simulink model "pendel_kartesisch"  (Simulink 7.0)
settings: Solver=ode45  StartTime=0.0  StopTime=tstop  FixedStep=0.3  MaxStep=0.25  RelTol=1e-6
values from neighbouring files (symbols this model uses):
  g = 9.81    [main_pendel_kartesisch.m]    (also in main_pendel_polar.m)
  l = 1    [main_pendel_kartesisch.m]    (also in main_pendel_polar.m)
  lamda_t0 = (vx0^2 + vy0^2 -g*y0)/(l^2)    [main_pendel_kartesisch.m]
  x0 = 1    [main_pendel_kartesisch.m]
  y0 = -sqrt(l^2-x0^2)    [main_pendel_kartesisch.m]
libraries: simulink x5
settings Model: Creator=adminus  LastModifiedBy=adminus
settings DataIOCC: OutputOption=SpecifiedOutputTimes  OutputTimes=[0:0.01:5]
settings OptimizationCC: BlockReduction=off
settings DebuggingCC: SaveWithParameterizedLinksMsg=none  SignalResolutionControl=TryResolveAllWithWarning  SolverPrmCheckMsg=none  MultiTaskDSMMsg=warning  MultiTaskCondExecSysMsg=none  StrictBusMsg=None
settings HardwareCC: TargetUnknown=on
settings RTWCC: IncludeERTFirstTime=on

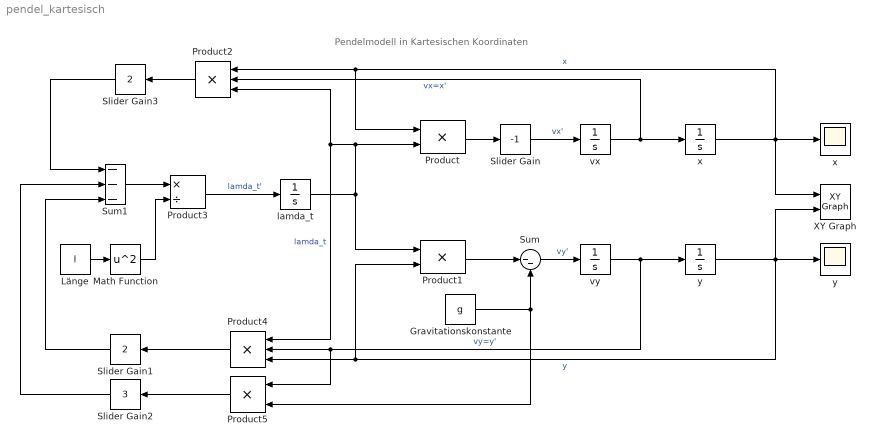
== system pendel_kartesisch ==
  note: Pendelmodell in Kartesischen Koordinaten
  Gravitationskonstante : Constant  Value=g
  Länge : Constant  Value=l
  Math Function : Math  Operator=square  SaturateOnIntegerOverflow=on
  Product : Product  SaturateOnIntegerOverflow=on  RndMeth=Zero  InputSameDT=on
  Product1 : Product  SaturateOnIntegerOverflow=on  RndMeth=Zero  InputSameDT=on
  Product2 : Product  Orientation=left  Inputs=3  SaturateOnIntegerOverflow=on  RndMeth=Zero  InputSameDT=on
  Product3 : Product  Inputs=*/  SaturateOnIntegerOverflow=on  RndMeth=Zero  InputSameDT=on
  Product4 : Product  Orientation=left  Inputs=3  SaturateOnIntegerOverflow=on  RndMeth=Zero  InputSameDT=on
  Product5 : Product  Orientation=left  SaturateOnIntegerOverflow=on  RndMeth=Zero  InputSameDT=on
  Slider Gain : simulink/Math Operations/Slider Gain  SystemSampleTime=-1  low=-1  gain=-1  high=2
  Slider Gain1 : simulink/Math Operations/Slider Gain  Orientation=left  SystemSampleTime=-1  low=-1  gain=2  high=2
  Slider Gain2 : simulink/Math Operations/Slider Gain  Orientation=left  SystemSampleTime=-1  low=-1  gain=3  high=3
  Slider Gain3 : simulink/Math Operations/Slider Gain  Orientation=left  SystemSampleTime=-1  low=-1  gain=2  high=2
  Sum : Sum  Inputs=|--  SaturateOnIntegerOverflow=on  InputSameDT=on
  Sum1 : Sum  Inputs=---  SaturateOnIntegerOverflow=on  InputSameDT=on
  XY Graph : simulink/Sinks/XY Graph  SystemSampleTime=-1  xmin=-1.1*l  xmax=1.1*l  ymin=-1.1*l  ymax=1.1*l  st=-1
  lamda_t : Integrator  InitialCondition=lamda_t0
  vx : Integrator
  vy : Integrator
  x : Scope
      settings: SaveName=ScopeData_v1_x
  "x " : Integrator  InitialCondition=x0
  y : Scope
      settings: SaveName=ScopeData_v1_y
  "y " : Integrator  InitialCondition=y0
  wires:
  lamda_t/1 -> Product/2, Product2/3, Product4/1, Product1/1  "lamda_t"
  Product1/1 -> Sum/1
  Slider Gain/1 -> vx/1  "vx'"
  Sum/1 -> vy/1  "vy'"
  Gravitationskonstante/1 -> Sum/2, Product5/2
  Sum1/1 -> Product3/1
  Länge/1 -> Math Function/1
  Product4/1 -> Slider Gain1/1
  Product2/1 -> Slider Gain3/1
  Product5/1 -> Slider Gain2/1
  Slider Gain1/1 -> Sum1/3
  Slider Gain2/1 -> Sum1/2
  Slider Gain3/1 -> Sum1/1
  "x "/1 -> Product/1, Product2/1, x/1, XY Graph/1  "x"
  Product/1 -> Slider Gain/1
  Product3/1 -> lamda_t/1  "lamda_t'"
  "y "/1 -> Product1/2, Product4/3, y/1, XY Graph/2  "y"
  vx/1 -> "x "/1, Product2/2  "vx=x'"
  vy/1 -> "y "/1, Product4/2, Product5/1  "vy=y'"
  Math Function/1 -> Product3/2
